simulink model "Lab2_2"  (Simulink 7.3)
settings: Solver=ode45  StartTime=1.0  StopTime=2.0  RelTol=1e-3
libraries: simulink x1
settings Model: Creator=Seva  LastModifiedBy=Seva

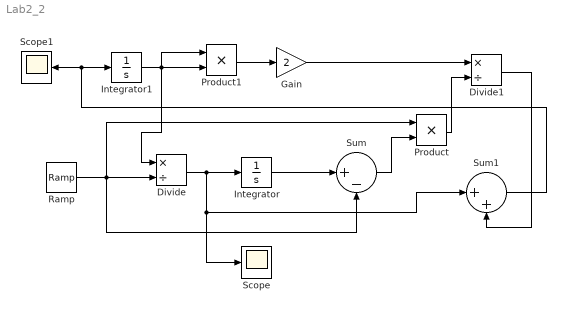
== system Lab2_2 ==
  Divide : Product  Inputs=*/  OutDataType=fixdt(1, 16)  OutScaling=2^-10
  Divide1 : Product  Inputs=*/  OutDataType=fixdt(1, 16)  OutScaling=2^-10
  Gain : Gain  Gain=2  ParameterDataType=fixdt(1, 16)  ParameterScaling=2^0  OutDataType=fixdt(1, 16)  OutScaling=2^0
  Integrator : Integrator
  Integrator1 : Integrator  InitialCondition=0.3
  Product : Product  OutDataType=fixdt(1, 16)  OutScaling=2^0  RndMeth=Zero
  Product1 : Product  OutDataType=fixdt(1, 16)  OutScaling=2^0  RndMeth=Zero
  Ramp : simulink/Sources/Ramp  SystemSampleTime=-1  slope=1  start=0  X0=0
  Scope : Scope
  Scope1 : Scope
  Sum : Sum  Inputs=|+-  OutDataType=fixdt(1, 16)  OutScaling=2^0
  Sum1 : Sum  Inputs=|++  OutDataType=fixdt(1, 16)  OutScaling=2^0
  wires:
  Divide/1 -> Integrator/1, Sum1/1, Scope/1
  Integrator/1 -> Sum/1
  Sum/1 -> Product/2
  Gain/1 -> Divide1/1
  Product/1 -> Divide1/2
  Divide1/1 -> Sum1/2
  Sum1/1 -> Integrator1/1, Scope1/1
  Integrator1/1 -> Product1/2, Product1/1, Divide/1
  Product1/1 -> Gain/1
  Ramp/1 -> Divide/2, Product/1, Sum/2
